simulink model "test_Simulator"  (R2021b)
settings: Solver=VariableStepAuto  StartTime=0.0  StopTime=10.0  RelTol=1e-3
settings Model: Creator=davide  LastModifiedBy=davide

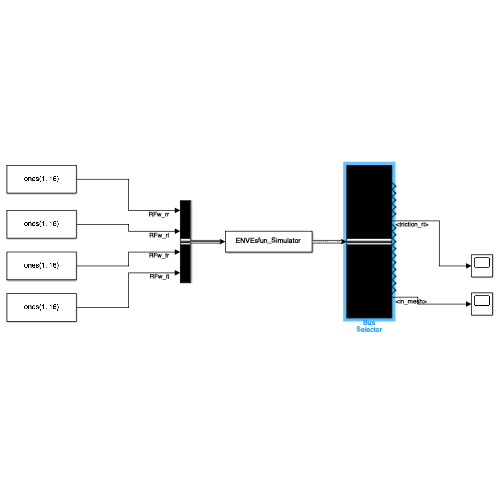
[thumbnail: Simulink's stored preview of the top-level diagram]
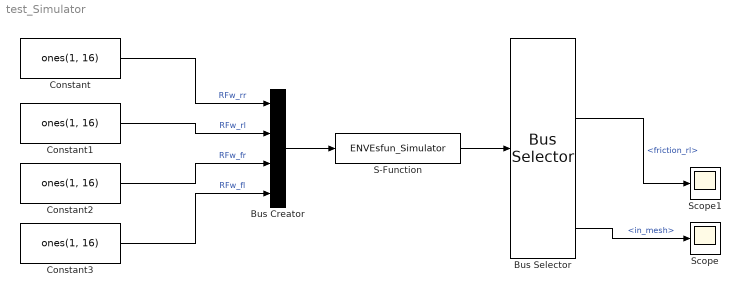
== system test_Simulator ==
  Bus Creator : BusCreator  Inputs=4  OutDataTypeStr=Bus: shellsRF
  Bus Selector : BusSelector  OutputSignals=RFpc_rr_ground,RFpc_rl_ground,RFpc_fr_ground,RFpc_fl_ground,friction_rr,friction_rl,friction_fr,friction_fl,rho_rr,rho_rl,rho_fr,rho_fl,rho_dot_rr,rho_dot_rl,rho_dot_fr,rho_dot_fl,in_mesh
  Constant{,1..3} (4 alike) : Constant  Value=ones(1, 16)
  S-Function : S-Function  FunctionName=ENVEsfun_Simulator  Parameters=p1, p2, p3, p4, p5, p6, p7, p8, p9, p10, p11, p12, p13, p14, p15  SFunctionDeploymentMode=off  EnableBusSupport=off
  Scope : Scope
  Scope1 : Scope
  wires:
  Bus Creator/1 -> S-Function/1
  S-Function/1 -> Bus Selector/1
  Constant/1 -> Bus Creator/1  "RFw_rr"
  Bus Selector/17 -> Scope/1  "<in_mesh>"
  Bus Selector/6 -> Scope1/1  "<friction_rl>"
  Constant3/1 -> Bus Creator/4  "RFw_fl"
  Constant2/1 -> Bus Creator/3  "RFw_fr"
  Constant1/1 -> Bus Creator/2  "RFw_rl"
